simulink model "L1"  (R2023b)
settings: Solver=VariableStepAuto  StartTime=0.0  StopTime=.04  RelTol=1e-3
libraries: spsRMSLib x6, spsVoltageMeasurementLib x4, eePowerMeasurement x3, spsSeriesRLCBranchLib x3, spsACVoltageSourceLib x2, spsCurrentMeasurementLib x2, spsGroundLib x2, spspowerguiLib x1
settings Model: Creator=offic  LastModifiedBy=offic
settings RTWCC: GPUComputeCapability=5.0

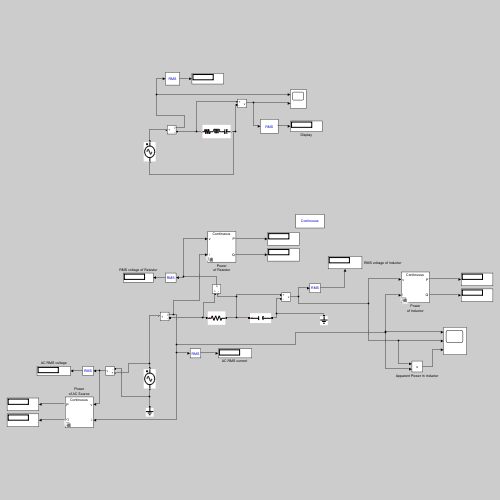
[thumbnail: Simulink's stored preview of the top-level diagram]
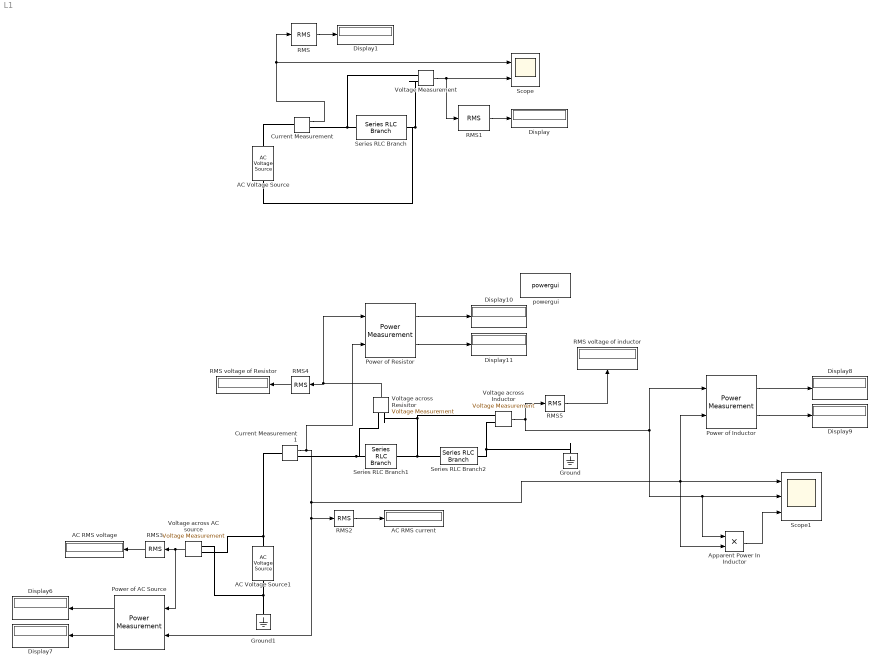
== system L1 ==
  "AC RMS current " : Display
  AC RMS voltage : Display
  AC Voltage Source : spsACVoltageSourceLib/AC Voltage Source  Amplitude=220  Phase=0  Frequency=50  SampleTime=0  Measurements=None  BusType=swing  Pref=10e3  Qref=0  Qmin=-inf  Qmax=+inf
  AC Voltage Source1 : spsACVoltageSourceLib/AC Voltage Source  Amplitude=220  Phase=0  Frequency=50  SampleTime=0  Measurements=None  BusType=swing  Pref=10e3  Qref=0  Qmin=-inf  Qmax=+inf
  Apparent Power In Inductor : Product
  Current Measurement : spsCurrentMeasurementLib/Current Measurement  PhasorSimulation=off  OutputType=Complex  PSBequivalent=0
  Current Measurement1 : spsCurrentMeasurementLib/Current Measurement  PhasorSimulation=off  OutputType=Complex  PSBequivalent=0
  Display{,1,6..11} (8 alike) : Display
      Display10 settings: Decimation=2
      Display11 settings: Decimation=2
      Display6 settings: Decimation=2
      Display7 settings: Decimation=2
      Display8 settings: Decimation=2
      Display9 settings: Decimation=2
  Ground : spsGroundLib/Ground  LConnTagsString=a
  Ground1 : spsGroundLib/Ground  LConnTagsString=a
  Power of AC Source : eePowerMeasurement/Power Measurement  LabelModeActiveChoice=Continuous  F=50  K=[1]  Ts=0
  Power of Inductor : eePowerMeasurement/Power Measurement  LabelModeActiveChoice=Continuous  F=50  K=[1]  Ts=0
  Power of Resistor : eePowerMeasurement/Power Measurement  LabelModeActiveChoice=Continuous  F=50  K=[1]  Ts=0
  RMS{,1..5} (6 alike) : spsRMSLib/RMS  TrueRMS=on  Freq=50  RMSInit=120  Ts=0
  RMS voltage of Resistor : Display
      settings: Decimation=2
  RMS voltage of inductor : Display
      settings: Decimation=2
  Scope : Scope  NumInputPorts=2
  Scope1 : Scope  NumInputPorts=3
  Series RLC Branch : spsSeriesRLCBranchLib/Series RLC Branch  LConnTagsString=__new0  RConnTagsString=__new0  BranchType=RLC  Resistance=1  Inductance=1e-3  SetiL0=off  InitialCurrent=0  Capacitance=1e-6  Setx0=off  InitialVoltage=0  Measurements=None
  Series RLC Branch1 : spsSeriesRLCBranchLib/Series RLC Branch  LConnTagsString=__new0  RConnTagsString=__new0  BranchType=R  Resistance=100  Inductance=1e-3  SetiL0=off  InitialCurrent=0  Capacitance=1e-6  Setx0=off  InitialVoltage=0  Measurements=None
  Series RLC Branch2 : spsSeriesRLCBranchLib/Series RLC Branch  LConnTagsString=__new0  RConnTagsString=__new0  BranchType=C  Resistance=1  Inductance=5e-1  SetiL0=off  InitialCurrent=0  Capacitance=1e-5  Setx0=off  InitialVoltage=0  Measurements=None
  Voltage Measurement : spsVoltageMeasurementLib/Voltage Measurement  PhasorSimulation=off  OutputType=Complex  PSBequivalent=0
  Voltage across AC source : spsVoltageMeasurementLib/Voltage Measurement  PhasorSimulation=off  OutputType=Complex  PSBequivalent=0
  Voltage across Inductor : spsVoltageMeasurementLib/Voltage Measurement  PhasorSimulation=off  OutputType=Complex  PSBequivalent=0
  Voltage across Resisitor : spsVoltageMeasurementLib/Voltage Measurement  PhasorSimulation=off  OutputType=Complex  PSBequivalent=0
  powergui : spspowerguiLib/powergui  Priority=1  SimulationMode=Continuous  SampleTime=50e-6  frequency=60  Iterations=50  frequencyindice=50  Pbase=100e6  ErrMax=1e-4  UnitsV=kV  UnitsW=MW  buscounter=0  FunctionMessages=off  echomessages=off  EnableUseOfTLC=off  CurrentSourceSwitches=off  DisableSnubberDevices=off  DisableRonSwitches=off  DisableVfSwitches=off  DisplayEquations=off  AutomaticDiscreteSolvers=off  SolverType=Tustin/Backward Euler (TBE)  Interpol=off  ExternalGateDelay=off  methode=off  Ts=100  x0status=blocks  SPID=on  SwTol=0  HookPort=off  NonlinearTolerance=1e-4  nMaxIteration=100  ContinueOnMaxIteration=off  RestoreLinks=warning  ResistiveCurrentMeasurement=off  Frange=[0:2:500]  Ylog=off  Xlog=on  ShowGrid=off  save=off  variable=ZData  structure=0  ZoomFFT=off  StartTime=0.0  cycles=1  DisplayStyle=1  fundamental=60  FreqAxis=off  MaxFrequency=1000  frequencyindicesteady=1  RmsSteady=1  display=off
  wires:
  Current Measurement/1 -> RMS/1, Scope/1
  RMS/1 -> Display1/1
  Voltage Measurement/1 -> RMS1/1, Scope/2
  RMS1/1 -> Display/1
  RMS2/1 -> "AC RMS current "/1
  Voltage across AC source/1 -> Power of AC Source/1, RMS3/1
  Voltage across Inductor/1 -> RMS5/1, Apparent Power In Inductor/1, Scope1/2, Power of Inductor/1
  Voltage across Resisitor/1 -> RMS4/1, Power of Resistor/1
  RMS5/1 -> RMS voltage of inductor/1
  RMS3/1 -> AC RMS voltage/1
  RMS4/1 -> RMS voltage of Resistor/1
  Power of AC Source/1 -> Display6/1
  Power of AC Source/2 -> Display7/1
  Power of Inductor/2 -> Display9/1
  Power of Inductor/1 -> Display8/1
  Power of Resistor/2 -> Display11/1
  Power of Resistor/1 -> Display10/1
  Current Measurement1/1 -> Scope1/1, Power of Inductor/2, Apparent Power In Inductor/2, Power of AC Source/2, RMS2/1, Power of Resistor/2
  Apparent Power In Inductor/1 -> Scope1/3
  connections:
  AC Voltage Source/RConn1 -- Current Measurement/LConn1
  Current Measurement/RConn1 -- Voltage Measurement/LConn1 -- Series RLC Branch/LConn1
  Voltage Measurement/LConn2 -- AC Voltage Source/LConn1 -- Series RLC Branch/RConn1
  Current Measurement1/RConn1 -- Voltage across Resisitor/LConn1 -- Series RLC Branch1/LConn1
  Current Measurement1/LConn1 -- Voltage across AC source/LConn1 -- AC Voltage Source1/RConn1
  Voltage across Inductor/LConn2 -- Ground/LConn1 -- Series RLC Branch2/RConn1
  Voltage across AC source/LConn2 -- AC Voltage Source1/LConn1 -- Ground1/LConn1
  Voltage across Inductor/LConn1 -- Voltage across Resisitor/LConn2 -- Series RLC Branch2/LConn1 -- Series RLC Branch1/RConn1
